simulink model "simPIFuzzy"  (R2023b)
settings: Solver=VariableStepAuto  StartTime=0.0  StopTime=initValues(2)  RelTol=1e-3
values from neighbouring files (symbols this model uses):
  initValues = initialize()    [Comparision.m]    (also in initialize.m = [T, tsim, stepValue, upperLim, lowerLim, K, tau])
  Ki = 2 / tp    (= 0.645161290323)    [cohenCoonPIVar.m]    (also in programClassic.m = Ki)
libraries: fuzblock x1
settings Model: Creator=usuario  LastModifiedBy=usuario
settings DataIOCC: ReturnWorkspaceOutputs=off

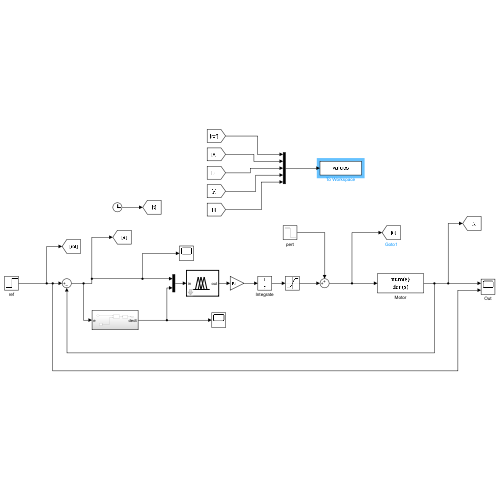
[thumbnail: Simulink's stored preview of the top-level diagram]
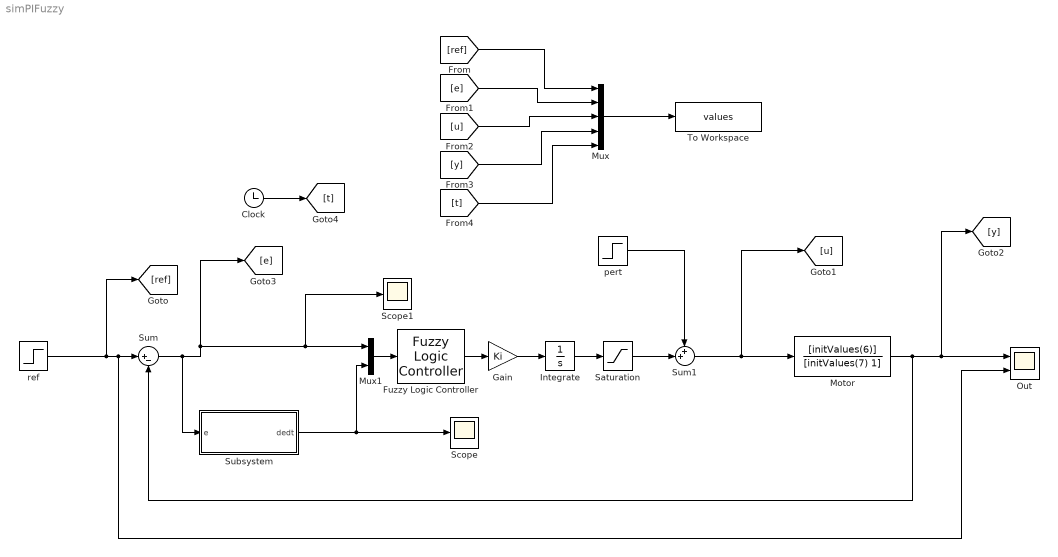
== system simPIFuzzy ==
  Clock : Clock
  Fuzzy Logic Controller : fuzblock/Fuzzy Logic  Controller  FIS='fuzzyPi.fis'  OutputSampleNumber=101  DataType=double  FuzzifiedInputs=off  RuleFiringStrengths=off  RuleOutputs=off  AggregatedOutputs=off  SimulateUsing=Interpreted execution  OutOfRangeInputValueMessage=warning  NoRuleFiredMessage=warning  EmptyOutputFuzzySetMessage=warning
  Gain : Gain  Gain=Ki
  Integrate : Integrator
  Motor : TransferFcn  Numerator=[initValues(6)]  Denominator=[initValues(7) 1]
  Mux : Mux  Inputs=5
  Mux1 : Mux  Inputs=2
  Out : Scope  NumInputPorts=2
  Saturation : Saturate  UpperLimit=initValues(4)  LowerLimit=initValues(5)
  Scope : Scope
  Scope1 : Scope
  Subsystem : Subsystem
  Sum : Sum  Inputs=|+-
  Sum1 : Sum  Inputs=++|
  To Workspace : ToWorkspace  VariableName=values  SaveFormat=Structure  SampleTime=initValues(1)
  pert : Step  Time=initValues(2)/2  After=-initValues(7)  SampleTime=0
  ref : Step  After=initValues(3)/2  SampleTime=0
  wires:
  Motor/1 -> Sum/2, [y], Out/1
  ref/1 -> [ref], Out/2, Sum/1
  [ref] -> Mux/1
  [y] -> Mux/4
  [e] -> Mux/2
  [u] -> Mux/3
  Mux/1 -> To Workspace/1
  Clock/1 -> [t]
  [t] -> Mux/5
  Mux1/1 -> Fuzzy Logic Controller/1
  Sum/1 -> Subsystem/1(e), Scope1/1, Mux1/1, [e]
  Integrate/1 -> Saturation/1
  Fuzzy Logic Controller/1 -> Gain/1
  Subsystem/1(dedt) -> Mux1/2, Scope/1
  Gain/1 -> Integrate/1
  Saturation/1 -> Sum1/2
  Sum1/1 -> [u], Motor/1
  pert/1 -> Sum1/1

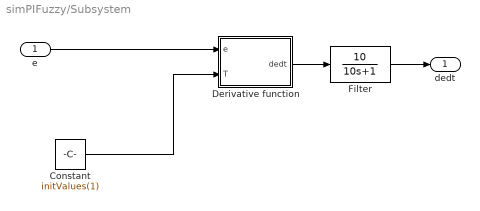
== system simPIFuzzy/Subsystem ==
  e : Inport
  Constant : Constant  Value=initValues(1)
  Derivative function : MATLAB Function  TreatAsAtomicUnit=on
  Filter : TransferFcn  Numerator=[10]  Denominator=[10 1]
  dedt : Outport
  wires:
  Constant/1 -> Derivative function/2(T)
  e/1 -> Derivative function/1(e)
  Derivative function/1(dedt) -> Filter/1
  Filter/1 -> dedt/1

== matlab function simPIFuzzy/Subsystem/Derivative function ==
  settings: updateMethod=DISCRETE  sampleTime=initValues(1)
  data: e input; dedt output; T input
function dedt = fcn(e, T)
    persistent pre_e;

    if isempty(pre_e)
        pre_e = e;
    end
    
    dedt = (pre_e - e)/T;
    pre_e = e;
end
